simulink model "Combined_Semi-Active_and_Passive"  (R2024a)
settings: Solver=VariableStepAuto  StartTime=0  StopTime=1372  RelTol=1e-3
undefined symbols (not defined in the file): sigbuilder_block
libraries: autolibshared x1
settings Model: SimulationMode=accelerator  Creator=LENOVO  LastModifiedBy=Jashwanth
settings SolverCC: AlgebraicLoopSolver=TrustRegion
settings DataIOCC: ReturnWorkspaceOutputs=off
settings DebuggingCC: MaxConsecutiveZCsMsg=none  UnconnectedInputMsg=warning  UnconnectedOutputMsg=warning  UnconnectedLineMsg=warning  ArithmeticOperatorsInVariantConditions=warning
settings ModelReferenceCC: EnableRefExpFcnMdlSchedulingChecks=on
settings SFSimCC: SimUseLocalCustomCode=off  CustomCodeUndefinedFunction=UseInterfaceOnly
settings RTWCC: RTWUseLocalCustomCode=off  GPUComputeCapability=3.5

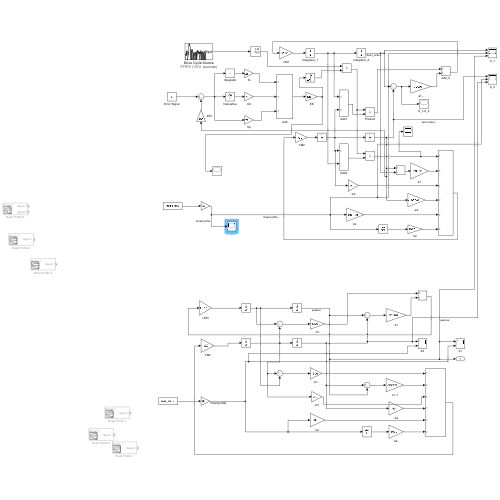
[thumbnail: Simulink's stored preview of the top-level diagram]
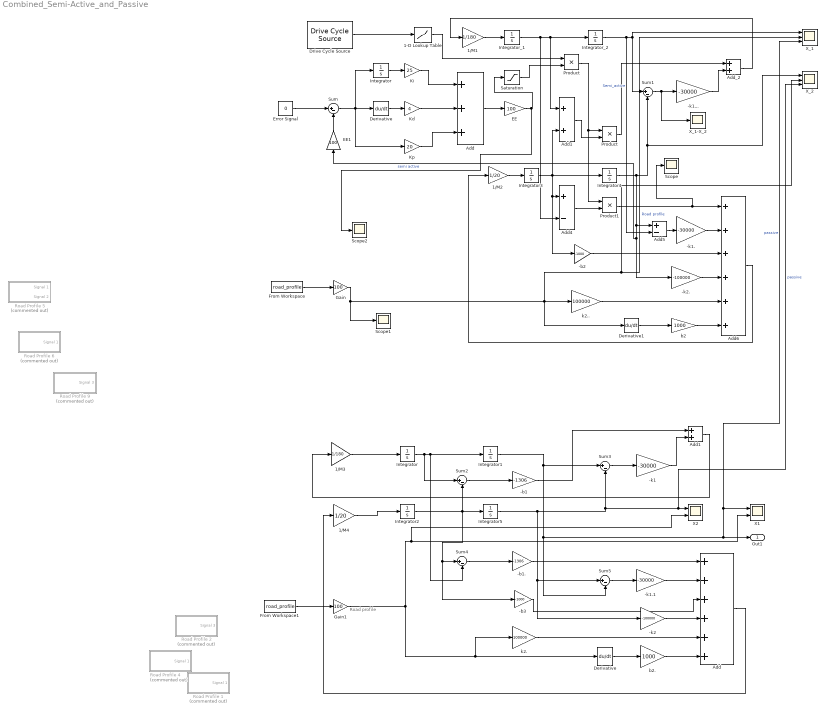
== system Combined_Semi-Active_and_Passive ==
  note: Road profile
  -b1 : Gain  Gain=-1306
  -b1. : Gain  Gain=-1306
  -b2 : Gain  Gain=-1000
  -b3 : Gain  Gain=-1000
  -k1 : Gain  Gain=-30000
  -k1. : Gain  Gain=-30000
  -k1... : Gain  Gain=-30000
  -k1.1 : Gain  Gain=-30000
  -k2 : Gain  Gain=-100000
  -k2. : Gain  Gain=-100000
  1-D Lookup Table : Lookup_n-D  NumberOfTableDimensions=1  BreakpointsForDimension1=[0 5.5 11.2 16.6 22.2]  Table=[900 1100 1306 1550 1700]  InternalRulePriority=Speed  RndMeth=Simplest
  1/M1 : Gain  Gain=1/180
  1/M2 : Gain  Gain=1/20
  1/M3 : Gain  Gain=1/180
  1/M4 : Gain  Gain=1/20
  Add : Sum  Inputs=++++++
  "Add " : Sum  Inputs=+++
  Add1 : Sum
  "Add1 " : Sum
  "Add4 " : Sum  Inputs=+-
  Add5 : Sum  Inputs=+-
  Add6 : Sum  Inputs=++++++
  Add_2 : Sum
  Derivative : Derivative
  "Derivative " : Derivative
  Derivative1 : Derivative
  Drive Cycle Source : autolibshared/Drive Cycle Source  cycleVar=FTP72  fileVar=cycleFTP75.mat  tfinal="1372  seconds"  cycleRepeat=off  outAccPort=off  outGearPort=off  gearList=No gear data  t_wot1=5  xdot_woto=0  xdot_wot1=30  t_wot2=20  xdot_wot2=0  t_wotend=30  srcUnit=m/s  outUnit=m/s  srcAccUnit=m/s/s  outAccUnit=m/s^2  dt=0  aMode=1  faultOption=off  velBnd=2  velBndUnit=mph  inUnit=m/s  timeBnd=1  failOption=off  stopSim=off  maxFaultCnt=10  maxFaultTime=2  maxTotFaultTime=15  traceOption=off  dtTrace=1  traceWindow=10  lastDCname=FTP72  lastOutUnit=mph  lastDT=0  lastTB=1  lastSB=2  forceCalcBound=off
  EE : Gain  Gain=100
  EE1 : Gain  Gain=100
  Error Signal : Constant  Value=0
  From Workspace : FromWorkspace  VariableName=road_profile  SampleTime=0.1
  From Workspace1 : FromWorkspace  VariableName=road_profile  SampleTime=0.1
  Gain : Gain  Gain=100
  Gain1 : Gain  Gain=100
  Integrator{,1..5} (6 alike) : Integrator
  "Integrator " : Integrator
  "Integrator_1 " : Integrator
  "Integrator_2 " : Integrator
  Kd : Gain  Gain=4
  Ki : Gain  Gain=25
  Kp : Gain  Gain=20
  Product : Product
  "Product " : Product
  Product1 : Product
  Road Profile 1 : Subsystem  Tag=STV Subsys  Commented=on  LoadFcn=sigbuilder_block('load');  StartFcn=sigbuilder_block('start');  StopFcn=sigbuilder_block('stop');  ClipboardFcn=sigbuilder_block('clipboard');  mask(Sigbuilder block){tuvar=[0:10]}
      mask help: Simulink:masks:SigbuilderBlock_MD
      mask init:
      | if ~strcmp(get_param(bdroot(gcbh),'SimulationStatus'),'stopped') tuvar = sigbuilder_block('maskInit'); end
      settings: CopyFcn=sigbuilder_block('copy');  DeleteFcn=sigbuilder_block('delete');  ModelCloseFcn=sigbuilder_block('modelClose');  PreSaveFcn=sigbuilder_block('preSave');  PauseFcn=sigbuilder_block('pause');  ContinueFcn=sigbuilder_block('continue');  NameChangeFcn=sigbuilder_block('namechange');  OpenFcn=sigbuilder_block('open',[6 0 1012.5 477.75 ]);  CloseFcn=sigbuilder_block('close');
      mask Display: plot(0, 0, 100, 100,[2, 2, 32, 32, 2], [68, 8, 8, 68, 68],[32, 2], [38, 38], [32, 19, 2],[53, 60, 44], [32, 17, 17, 2],[16, 16, 31, 31]);txt = getActiveGroup(gcbh);text(2, 100, txt,'verticalAlignment', 'top');
  Road Profile 2 : Subsystem  Tag=STV Subsys  Commented=on  LoadFcn=sigbuilder_block('load');  StartFcn=sigbuilder_block('start');  StopFcn=sigbuilder_block('stop');  ClipboardFcn=sigbuilder_block('clipboard');  mask(Sigbuilder block){tuvar=[0:10]}
      mask help: Simulink:masks:SigbuilderBlock_MD
      mask init:
      | if ~strcmp(get_param(bdroot(gcbh),'SimulationStatus'),'stopped') tuvar = sigbuilder_block('maskInit'); end
      settings: CopyFcn=sigbuilder_block('copy');  DeleteFcn=sigbuilder_block('delete');  ModelCloseFcn=sigbuilder_block('modelClose');  PreSaveFcn=sigbuilder_block('preSave');  PauseFcn=sigbuilder_block('pause');  ContinueFcn=sigbuilder_block('continue');  NameChangeFcn=sigbuilder_block('namechange');  OpenFcn=sigbuilder_block('open',[141 130.2 550.5 359.55 ]);  CloseFcn=sigbuilder_block('close');
      mask Display: plot(0, 0, 100, 100,[2, 2, 32, 32, 2], [68, 8, 8, 68, 68],[32, 2], [38, 38], [32, 19, 2],[53, 60, 44], [32, 17, 17, 2],[16, 16, 31, 31]);txt = getActiveGroup(gcbh);text(2, 100, txt,'verticalAlignment', 'top');
  Road Profile 4 : Subsystem  Tag=STV Subsys  Commented=on  LoadFcn=sigbuilder_block('load');  StartFcn=sigbuilder_block('start');  StopFcn=sigbuilder_block('stop');  ClipboardFcn=sigbuilder_block('clipboard');  mask(Sigbuilder block){tuvar=[0:10]}
      mask help: Simulink:masks:SigbuilderBlock_MD
      mask init:
      | if ~strcmp(get_param(bdroot(gcbh),'SimulationStatus'),'stopped') tuvar = sigbuilder_block('maskInit'); end
      settings: CopyFcn=sigbuilder_block('copy');  DeleteFcn=sigbuilder_block('delete');  ModelCloseFcn=sigbuilder_block('modelClose');  PreSaveFcn=sigbuilder_block('preSave');  PauseFcn=sigbuilder_block('pause');  ContinueFcn=sigbuilder_block('continue');  NameChangeFcn=sigbuilder_block('namechange');  OpenFcn=sigbuilder_block('open',[6 0 1012.5 477.75 ]);  CloseFcn=sigbuilder_block('close');
      mask Display: plot(0, 0, 100, 100,[2, 2, 32, 32, 2], [68, 8, 8, 68, 68],[32, 2], [38, 38], [32, 19, 2],[53, 60, 44], [32, 17, 17, 2],[16, 16, 31, 31]);txt = getActiveGroup(gcbh);text(2, 100, txt,'verticalAlignment', 'top');
  Road Profile 5 : Subsystem  Tag=STV Subsys  Commented=on  LoadFcn=sigbuilder_block('load');  StartFcn=sigbuilder_block('start');  StopFcn=sigbuilder_block('stop');  ClipboardFcn=sigbuilder_block('clipboard');  mask(Sigbuilder block){tuvar=[0:10]}
      mask help: Simulink:masks:SigbuilderBlock_MD
      mask init:
      | if ~strcmp(get_param(bdroot(gcbh),'SimulationStatus'),'stopped') tuvar = sigbuilder_block('maskInit'); end
      settings: CopyFcn=sigbuilder_block('copy');  DeleteFcn=sigbuilder_block('delete');  ModelCloseFcn=sigbuilder_block('modelClose');  PreSaveFcn=sigbuilder_block('preSave');  PauseFcn=sigbuilder_block('pause');  ContinueFcn=sigbuilder_block('continue');  NameChangeFcn=sigbuilder_block('namechange');  OpenFcn=sigbuilder_block('open',[5.4 36 1141.2 516.6 ]);  CloseFcn=sigbuilder_block('close');
      mask Display: plot(0, 0, 100, 100,[2, 2, 32, 32, 2], [68, 8, 8, 68, 68],[32, 2], [38, 38], [32, 19, 2],[53, 60, 44], [32, 17, 17, 2],[16, 16, 31, 31]);txt = getActiveGroup(gcbh);text(2, 100, txt,'verticalAlignment', 'top');
  Road Profile 6 : Subsystem  Tag=STV Subsys  Commented=on  LoadFcn=sigbuilder_block('load');  StartFcn=sigbuilder_block('start');  StopFcn=sigbuilder_block('stop');  ClipboardFcn=sigbuilder_block('clipboard');  mask(Sigbuilder block){tuvar=[0:10]}
      mask help: Simulink:masks:SigbuilderBlock_MD
      mask init:
      | if ~strcmp(get_param(bdroot(gcbh),'SimulationStatus'),'stopped') tuvar = sigbuilder_block('maskInit'); end
      settings: CopyFcn=sigbuilder_block('copy');  DeleteFcn=sigbuilder_block('delete');  ModelCloseFcn=sigbuilder_block('modelClose');  PreSaveFcn=sigbuilder_block('preSave');  PauseFcn=sigbuilder_block('pause');  ContinueFcn=sigbuilder_block('continue');  NameChangeFcn=sigbuilder_block('namechange');  OpenFcn=sigbuilder_block('open',[6 0 1012.5 477.75 ]);  CloseFcn=sigbuilder_block('close');
      mask Display: plot(0, 0, 100, 100,[2, 2, 32, 32, 2], [68, 8, 8, 68, 68],[32, 2], [38, 38], [32, 19, 2],[53, 60, 44], [32, 17, 17, 2],[16, 16, 31, 31]);txt = getActiveGroup(gcbh);text(2, 100, txt,'verticalAlignment', 'top');
  Road Profile 9 : Subsystem  Tag=STV Subsys  Commented=on  LoadFcn=sigbuilder_block('load');  StartFcn=sigbuilder_block('start');  StopFcn=sigbuilder_block('stop');  ClipboardFcn=sigbuilder_block('clipboard');  mask(Sigbuilder block){tuvar=[0:10]}
      mask help: Simulink:masks:SigbuilderBlock_MD
      mask init:
      | if ~strcmp(get_param(bdroot(gcbh),'SimulationStatus'),'stopped') tuvar = sigbuilder_block('maskInit'); end
      settings: CopyFcn=sigbuilder_block('copy');  DeleteFcn=sigbuilder_block('delete');  ModelCloseFcn=sigbuilder_block('modelClose');  PreSaveFcn=sigbuilder_block('preSave');  PauseFcn=sigbuilder_block('pause');  ContinueFcn=sigbuilder_block('continue');  NameChangeFcn=sigbuilder_block('namechange');  OpenFcn=sigbuilder_block('open',[141 130.2 550.5 359.55 ]);  CloseFcn=sigbuilder_block('close');
      mask Display: plot(0, 0, 100, 100,[2, 2, 32, 32, 2], [68, 8, 8, 68, 68],[32, 2], [38, 38], [32, 19, 2],[53, 60, 44], [32, 17, 17, 2],[16, 16, 31, 31]);txt = getActiveGroup(gcbh);text(2, 100, txt,'verticalAlignment', 'top');
  Saturation : Saturate  UpperLimit=1  LowerLimit=-1
  Scope : Scope
  Scope1 : Scope
  Scope2 : Scope
  Sum{,1..5} (6 alike) : Sum  Inputs=|+-
  X1 : Scope  NumInputPorts=2
  X2 : Scope  NumInputPorts=2
  X_1 : Scope  NumInputPorts=3
  X_1-X_2 : Scope
  X_2 : Scope  NumInputPorts=3
  b2 : Gain  Gain=1000
  b2. : Gain  Gain=1000
  k2. : Gain  Gain=100000
  k2.. : Gain  Gain=100000
  Out1 : Outport  VectorParamsAs1DForOutWhenUnconnected=off
  wires:
  "Integrator "/1 -> Ki/1
  "Derivative "/1 -> Kd/1
  Kp/1 -> "Add "/3
  Kd/1 -> "Add "/2
  Ki/1 -> "Add "/1
  Sum/1 -> Kp/1, "Integrator "/1, "Derivative "/1
  "Add "/1 -> EE/1
  EE/1 -> Scope2/1, Saturation/1
  Saturation/1 -> Product/2
  1/M1/1 -> "Integrator_1 "/1
  "Integrator_1 "/1 -> "Add4 "/2, "Add1 "/1, "Integrator_2 "/1
  "Integrator_2 "/1 -> Add5/2, X_1/1, Sum1/1  "Semi_active"
  -k1.../1 -> Add_2/2
  Sum1/1 -> -k1.../1, X_1-X_2/1
  1/M2/1 -> Integrator3/1
  Integrator4/1 -> Sum1/2, X_2/1, Add5/1, EE1/1, -k2./1  "semi active"
  Integrator3/1 -> "Add1 "/2, Integrator4/1, -b2/1, "Add4 "/1
  "Add4 "/1 -> Product1/2
  Product/1 -> "Product "/1, Product1/1
  Add_2/1 -> 1/M1/1
  Product1/1 -> Scope/1, Add6/1
  -k1./1 -> Add6/2
  Add5/1 -> -k1./1
  -k2./1 -> Add6/4
  -b2/1 -> Add6/3
  "Add1 "/1 -> "Product "/2
  Derivative1/1 -> b2/1
  b2/1 -> Add6/6
  k2../1 -> Add6/5
  From Workspace/1 -> Gain/1
  "Product "/1 -> Add_2/1
  Add6/1 -> 1/M2/1
  Error Signal/1 -> Sum/1
  EE1/1 -> Sum/2
  Add1/1 -> 1/M3/1
  Integrator/1 -> Sum2/1, Sum4/2, Integrator1/1
  -b1./1 -> Add/1
  Sum4/1 -> -b1./1
  k2./1 -> Add/5
  b2./1 -> Add/6
  Derivative/1 -> b2./1
  -k2/1 -> Add/4
  -k1/1 -> Add1/2
  Add/1 -> 1/M4/1
  From Workspace1/1 -> Gain1/1
  Integrator1/1 -> Sum3/1, X_1/3, X1/1, Out1/1, Sum5/2  "passive"
  Sum3/1 -> -k1/1
  -b3/1 -> Add/3
  Sum2/1 -> -b1/1
  -k1.1/1 -> Add/2
  -b1/1 -> Add1/1
  Integrator5/1 -> Sum5/1, -k2/1, Sum3/2, X_2/3, X2/1  "passive"
  Sum5/1 -> -k1.1/1
  Integrator2/1 -> Sum4/1, -b3/1, Sum2/2, Integrator5/1
  1/M4/1 -> Integrator2/1
  1/M3/1 -> Integrator/1
  1-D Lookup Table/1 -> Product/1
  Drive Cycle Source/1 -> 1-D Lookup Table/1
  Gain/1 -> Scope1/1, Derivative1/1, X_2/2, X_1/2, k2../1  "Road profile"
  Gain1/1 -> Derivative/1, k2./1, X2/2, X1/2

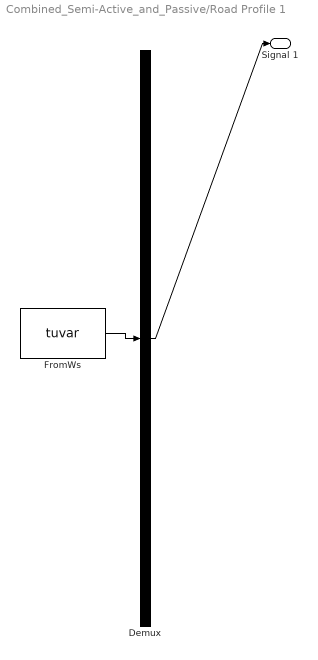
== system Combined_Semi-Active_and_Passive/Road Profile 1 ==
  Demux : Demux  Tag=STV Demux  Outputs=1
      settings: DisplayOption=none
  FromWs : FromWorkspace  Tag=STV FromWs  VariableName=tuvar
      SigBuilderData=|
      | common.afterFinalStr = 'Extrapolate'
      | common.sampleTime = 0
      | dataSet.timeRange = [0 40]
      | dataSet.name = 'Group 1'
      | sbobj.Groups.Name = 'Group 1'
      | sbobj.Groups.Signals.Name = 'Signal 1'
      | sbobj.Groups.Signals.XData = [0 2 3 4 5 7 10 11 12 13 14 15 16 17 18 19 20 21 22 23 24 25 26 27 28 29 30 31 32 33 34 35 36 37 38 40]
      | sbobj.Groups.Signals.YData = [0 0 0 0 0 0.1 0 0 0 0 0 0 0 0 0 0 0 0 0 0 0 0 0 0 0 0 0 0 0 0 0 0 0 0 0 0]
      | sbobj.Groups.TimeRange = [0 40]
  Signal 1 : Outport  Tag=STV Outport  VectorParamsAs1DForOutWhenUnconnected=off
  wires:
  FromWs/1 -> Demux/1
  Demux/1 -> Signal 1/1

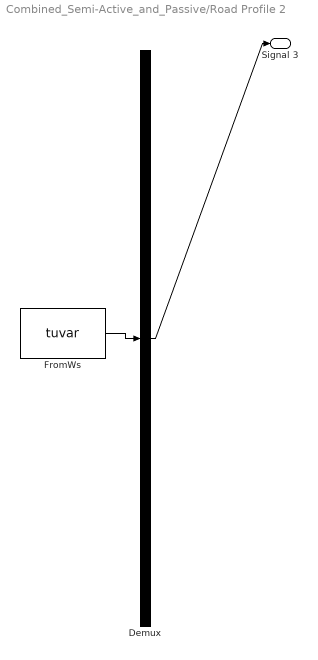
== system Combined_Semi-Active_and_Passive/Road Profile 2 ==
  Demux : Demux  Tag=STV Demux  Outputs=1
      settings: DisplayOption=none
  FromWs : FromWorkspace  Tag=STV FromWs  VariableName=tuvar
      SigBuilderData=|
      | common.afterFinalStr = 'Extrapolate'
      | common.sampleTime = 0
      | dataSet.timeRange = [0 5]
      | dataSet.name = 'Group 1'
      | sbobj.Groups.Name = 'Group 1'
      | sbobj.Groups.Signals.Name = 'Signal 3'
      | sbobj.Groups.Signals.XData = [0 0.2 0.3 0.4 0.5 0.6 0.8 0.9 1 1.1 1.2 1.3 1.4 1.5 1.6 1.7 1.8 1.9 2 2.1 2.2 2.3 2.4 2.5 2.6 2.7 2.8 2.9 3 3.2 3.4 3.5 3.6 3.7 3.8 3.9 4 4.1 4.2 4.3 4.4 4.5 4.6 4.7 4.8 4.9 5]
      | sbobj.Groups.Signals.YData = [0 0 0 0 0 0.1 0 0 0 0 0 0 0 0 0 0 0 0 0 0 0 0 0 0 0 0 0 0 0 0.05 0 0 0 0 0 0 0 0 0 0 0 0 0 0 0 0 0]
      | sbobj.Groups.TimeRange = [0 5]
  Signal 3 : Outport  Tag=STV Outport  VectorParamsAs1DForOutWhenUnconnected=off
  wires:
  FromWs/1 -> Demux/1
  Demux/1 -> Signal 3/1

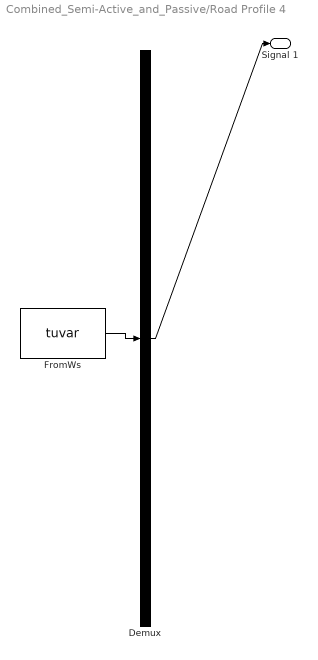
== system Combined_Semi-Active_and_Passive/Road Profile 4 ==
  Demux : Demux  Tag=STV Demux  Outputs=1
      settings: DisplayOption=none
  FromWs : FromWorkspace  Tag=STV FromWs  VariableName=tuvar
      SigBuilderData=|
      | common.afterFinalStr = 'Extrapolate'
      | common.sampleTime = 0
      | dataSet.timeRange = [0 40]
      | dataSet.name = 'Group 1'
      | sbobj.Groups.Name = 'Group 1'
      | sbobj.Groups.Signals.Name = 'Signal 1'
      | sbobj.Groups.Signals.XData = [0 2 3 4 5 6 7 8 9 10 11 12 13 14 15 16 17 18 19 20 21 22 23 24 25 26 27 28 29 30 31 32 33 34 35 36 37 38 40]
      | sbobj.Groups.Signals.YData = [0 0 0 0 0 0.083 0.1 0.09 0.06 0 0 0 0 0 0 0 0 0 0 0 0 0 0 0 0 0 0 0 0 0 0 0 0 0 0 0 0 0 0]
      | sbobj.Groups.TimeRange = [0 40]
  Signal 1 : Outport  Tag=STV Outport  VectorParamsAs1DForOutWhenUnconnected=off
  wires:
  FromWs/1 -> Demux/1
  Demux/1 -> Signal 1/1

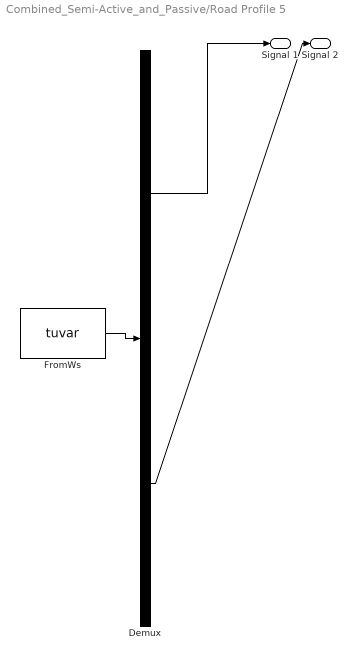
== system Combined_Semi-Active_and_Passive/Road Profile 5 ==
  Demux : Demux  Tag=STV Demux  Outputs=2
      settings: DisplayOption=none
  FromWs : FromWorkspace  Tag=STV FromWs  VariableName=tuvar
      SigBuilderData=|
      | common.afterFinalStr = 'Extrapolate'
      | common.sampleTime = 0
      | dataSet.timeRange = [0 40]
      | dataSet.name = 'Group 1'
      | sbobj.Groups.Name = 'Group 1'
      | sbobj.Groups.Signals(1).Name = 'Signal 1'
      | sbobj.Groups.Signals(1).XData = [0 2 3 4 5 6 7 8 9 10 11 12 13 14 15 16 17 18 19 20 21 22 23 24 25 26 27 28 29 30 31 32 33 34 35 36 37 38 40]
      | sbobj.Groups.Signals(1).YData = [0 0 0 0 0 0.083 0.1 0.09 0.06 0 0 0 0 0 0 0 0 0 0 0 0 0 0 0 0 0 0 0 0 0 0 0 0 0 0 0 0 0 0]
      | sbobj.Groups.Signals(2).Name = 'Signal 2'
      | sbobj.Groups.Signals(2).XData = [0 40]
      | sbobj.Groups.Signals(2).YData = [0.49 0.49]
      | sbobj.Groups.TimeRange = [0 40]
  Signal 1 : Outport  Tag=STV Outport  VectorParamsAs1DForOutWhenUnconnected=off
  Signal 2 : Outport  Tag=STV Outport  Port=2
  wires:
  FromWs/1 -> Demux/1
  Demux/1 -> Signal 1/1
  Demux/2 -> Signal 2/1

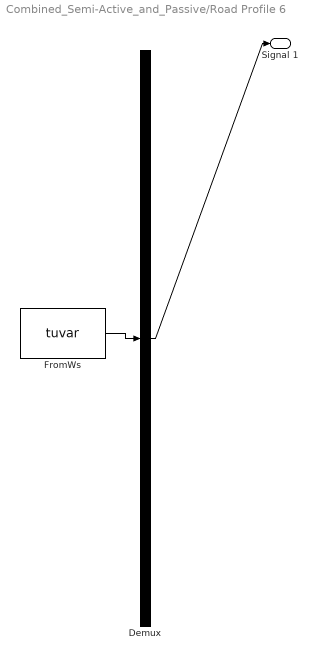
== system Combined_Semi-Active_and_Passive/Road Profile 6 ==
  Demux : Demux  Tag=STV Demux  Outputs=1
      settings: DisplayOption=none
  FromWs : FromWorkspace  Tag=STV FromWs  VariableName=tuvar
      SigBuilderData=|
      | common.afterFinalStr = 'Extrapolate'
      | common.sampleTime = 0
      | dataSet.timeRange = [0 40]
      | dataSet.name = 'Group 1'
      | sbobj.Groups.Name = 'Group 1'
      | sbobj.Groups.Signals.Name = 'Signal 1'
      | sbobj.Groups.Signals.XData = [0 2 3 4 5 7 10 11 12 13 14 15 16 17 18 19 20 21 22 23 24 25 26 27 28 29 30 31 32 33 34 35 36 37 38 40]
      | sbobj.Groups.Signals.YData = [0 0 0 0 0 0.1 0 0 0 0 0 0 0 0 0 0 0 0 0 0 0 0 0 0 0 0 0 0 0 0 0 0 0 0 0 0]
      | sbobj.Groups.TimeRange = [0 40]
  Signal 1 : Outport  Tag=STV Outport  VectorParamsAs1DForOutWhenUnconnected=off
  wires:
  FromWs/1 -> Demux/1
  Demux/1 -> Signal 1/1

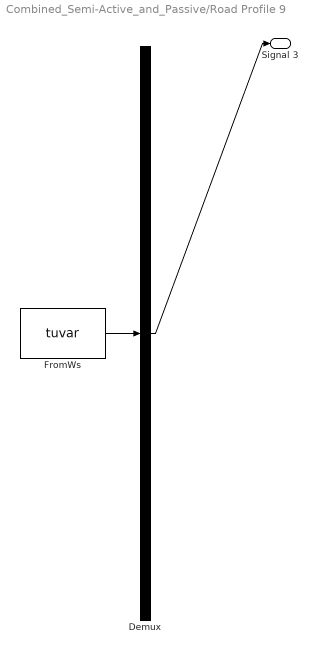
== system Combined_Semi-Active_and_Passive/Road Profile 9 ==
  Demux : Demux  Tag=STV Demux  Outputs=1
      settings: DisplayOption=none
  FromWs : FromWorkspace  Tag=STV FromWs  VariableName=tuvar
      SigBuilderData=|
      | common.afterFinalStr = 'Extrapolate'
      | common.sampleTime = 0
      | dataSet.timeRange = [0 40]
      | dataSet.name = 'Group 1'
      | sbobj.Groups.Name = 'Group 1'
      | sbobj.Groups.Signals.Name = 'Signal 3'
      | sbobj.Groups.Signals.XData = [0 5 5 40]
      | sbobj.Groups.Signals.YData = [0 0 0.1 0.1]
      | sbobj.Groups.TimeRange = [0 40]
  Signal 3 : Outport  Tag=STV Outport  VectorParamsAs1DForOutWhenUnconnected=off
  wires:
  FromWs/1 -> Demux/1
  Demux/1 -> Signal 3/1
